simulink model "cst_robotarm_optimized"  (R2024b)
settings: Solver=ode23t  StartTime=0.0  StopTime=5  FixedStep=0.0001  MaxStep=0.05  RelTol=1e-3  EnableMultiTasking=on
model workspace (MAT data in the model file):
  DCMotor_J = 0.0946866703633
  DCMotor_K = 0.477771340295
  DCMotor_Kf = 0.921434142151
  DCMotor_L = 0.000316454712175
  DCMotor_R = 4.99938152603
  Ts = 0.1
  dFilt = [1 -0.1202]
  nFilt = [0.4399 0.4399]
values from neighbouring files (symbols this model uses):
  m = s(1)    [PIDOptimizer.m]    (also in cost.m; cost_adapted.m; cost_adopted.m)
  s = size(signals)    [PIDOptimizer.m]    (also in cost.m; cost_adapted.m; cost_adopted.m)
undefined symbols (not defined in the file or in its folder): joint1_ctrl, joint2_ctrl, joint3_ctrl, joint4_ctrl, joint5_ctrl, joint6_ctrl, X, Y, Z
libraries: sm_lib x244, fl_lib x75, nesl_utility x28, ee_lib x21, slpidlib x6, SignalEditorBlockLib x1
(part 1 of 7)
settings Model: SimulationMode=accelerator  Creator=The MathWorks, Inc.  LastModifiedBy=sergi
settings SolverCC: AlgebraicLoopSolver=TrustRegion
settings DataIOCC: LimitDataPoints=on  SaveFormat=Array  InspectSignalLogs=on  SaveTime=off  ReturnWorkspaceOutputs=off
settings OptimizationCC: ReuseModelBlockBuffer=off  ExpressionDepthLimit=2147483647  LifeSpan=inf
settings DebuggingCC: UnderspecifiedInitializationDetection=Classic  MergeDetectMultiDrivingBlocksExec=none  FcnCallInpInsideContextMsg=warning  UnconnectedInputMsg=warning  UnconnectedOutputMsg=warning  UnconnectedLineMsg=warning  StateNameClashWarn=warning  SFUnexpectedBacktrackingDiag=warning  SFNoUnconditionalDefaultTransitionDiag=warning  SFExecutionAtInitializationDiag=none  ArithmeticOperatorsInVariantConditions=warning
settings HardwareCC: ProdBitPerPointer=32  ProdBitPerSizeT=32  ProdBitPerPtrDiffT=32  ProdLargestAtomicFloat=None  ProdIntDivRoundTo=Undefined  ProdEndianess=Unspecified  ProdWordSize=32  ProdHWDeviceType=32-bit Generic
settings ModelReferenceCC: EnableRefExpFcnMdlSchedulingChecks=on  PropagateSignalLabelsOutOfModel=off
settings SFSimCC: SimUseLocalCustomCode=off  CustomCodeUndefinedFunction=UseInterfaceOnly
settings RTWCC: RTWUseLocalCustomCode=off  GPUComputeCapability=3.5
settings CodeAppCC: StateflowObjectComments=on
settings GRTTargetCC: TargetLangStandard=C89/C90 (ANSI)  CombineOutputUpdateFcns=off  GRTInterface=on
settings ConfigComp: CovMetricSettings=dw  CovSaveCumulativeToWorkspaceVar=on  CovSaveSingleToWorkspaceVar=on  CovExternalEMLEnable=off  CovSFcnEnable=off
settings SimscapeCC: SimscapeNormalizeSystem=off
settings ConfigurationSet: Description=SimMechanics 2G
settings DiagnosticsConfigSet: SimMechanicsUnconnectedFramePorts=none
settings ExplorerConfigSet: InternalSimMechanicsExplorerSettings="<ExplorerConfiguration><canonicalview>planar_xy</canonicalview><AnimationSetting><BasePlaybackSpeed>1.0</BasePlaybackSpeed><PlaybackSpeedFactor>1.0</PlaybackSpeedFactor></AnimationSetting><TilePanel><TileInfo><Tiles Columns=\"1\" Count=\"1\" Rows=\"1\"><Column Left=\"2\" Weight=\"1\"/><Column Left=\"708\"/><Row Top=\"2\" Weight=\"1\"/><Row Top=\"595\"/><Tile Height=\"1\" Width=\"1\" X=\"0\" Y=\"0\"/></Tiles></TileInfo><SceneInfo><SceneViewer><BGColor><R>0.80000001192092896</R><G>0.80000001192092896</G><B>0.80000001192092896</B></BGColor><Camera><Position><X>0.30752487944302698</X><Y>0.57922836563106395</Y><Z>0.35651305744246536</Z></Position><Center><X>-0.033772386749033274</X><Y>0.23793109943898419</Y><Z>0.015215791250393121</Z></Center><Up><X>-0.40824829046386307</X><Y>0.81649658092772615</Y><Z>-0.40824829046386307</Z></Up><Left>-0.063283674940751766</Left><Right>0.063283674940751766</Right><Bottom>-0.22321517040744418</Bottom><Top>0.22321517040744418</Top></Camera></SceneViewer></SceneInfo></TilePanel></ExplorerConfiguration>"

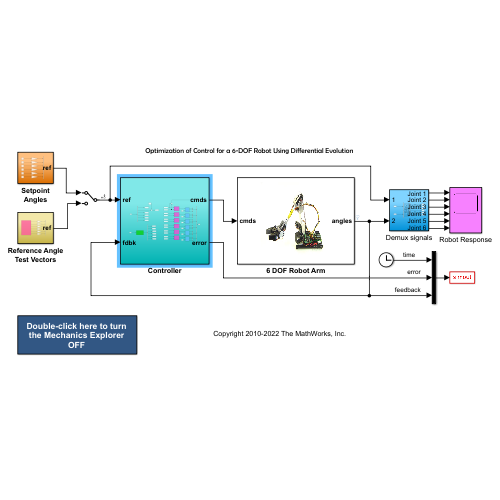
[thumbnail: Simulink's stored preview of the top-level diagram]
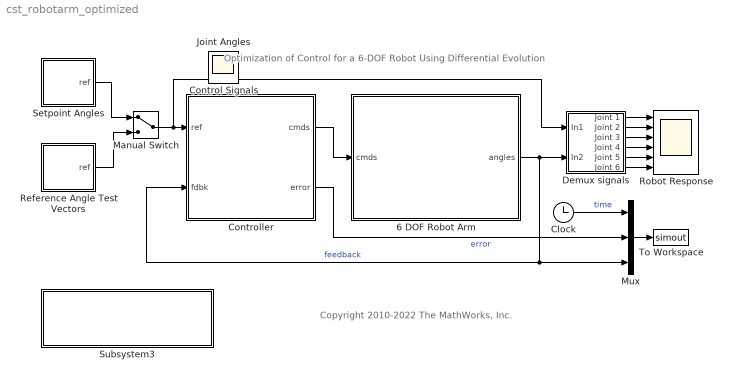
== system cst_robotarm_optimized ==
  note: Optimization of Control for a 6-DOF Robot Using Differential Evolution
  note: Copyright 2010-2022 The MathWorks, Inc.
  6 DOF Robot Arm : Subsystem
      mask Display: image('RobotArmSystem.jpg',[0.2 0.05 0.6 0.9])
  Clock : Clock
  Controller : Subsystem
  Demux signals : Subsystem
  Manual Switch : ManualSwitch
  Mux : Mux  Inputs=3
  Reference Angle Test Vectors : Subsystem
  Robot Response : Scope  NumInputPorts=6
  Setpoint Angles : Subsystem
  Subsystem3 : Subsystem
      mask init:
      | % Get current simulation mode
      | vizStatus = get_param(gcs,'SimMechanicsOpenEditorOnUpdate');
      | 
      | if strcmp(vizStatus,'on')
      |     viz = 'OFF';
      | else
      |     viz = 'ON';
      | end
      settings: OpenFcn=|
      | % Get current SimMechanics Explorer status
      | vizStatus = get_param(gcs ,'SimMechanicsOpenEditorOnUpdate');
      | 
      | if strcmp(vizStatus,'on')
      | % Set SimMechanics Explorer status to OFF
      |      set_param(gcs,'SimMechanicsOpenEditorOnUpdate','off');
      |      set_param(gcb,'BackgroundColor','[0.4706, 0.4706, 0.4706]');
      |      set_param(gcs,'SimulationCommand','update');
      | else
      | % Set SimMechanics Explorer status to ON
      |      set_param(gcs,'SimMechanicsOpenEditorOnUpdate','on');
      |      set_param(gcb,'BackgroundColor','[0.1961, 0.3412, 0.5176]')
      |      set_param(gcs,'SimulationCommand','update');
      | end
      mask Display:
      | color('white')
      | text(0.5,0.65,'Double-click here to turn\nthe Mechanics Explorer',...
      |     'horizontalAlignment','center',...
      |     'verticalAlignment','middle');
      | text(0.5,0.25,viz,...
      |     'horizontalAlignment','center',...
      |     'verticalAlignment','middle')
  To Workspace : ToWorkspace  VariableName=simout  SaveFormat=Structure With Time  SampleTime=-1
  Control Signals : Scope
  Joint Angles : Scope
  wires:
  Controller/1(cmds) -> 6 DOF Robot Arm/1(cmds)
  Manual Switch/1 -> Demux signals/1(In1), Controller/1(ref)
  Reference Angle Test Vectors/1(ref) -> Manual Switch/2
  Setpoint Angles/1(ref) -> Manual Switch/1
  Mux/1 -> To Workspace/1
  Clock/1 -> Mux/1  "time"
  6 DOF Robot Arm/1(angles) -> Mux/3, Controller/2(fdbk), Demux signals/2(In2)  "feedback"
  Controller/2(error) -> Mux/2  "error"
  Demux signals/1(Joint 1) -> Robot Response/1
  Demux signals/2(Joint 2) -> Robot Response/2
  Demux signals/3(Joint 3) -> Robot Response/3
  Demux signals/4(Joint 4) -> Robot Response/4
  Demux signals/5(Joint 5) -> Robot Response/5
  Demux signals/6(Joint 6) -> Robot Response/6

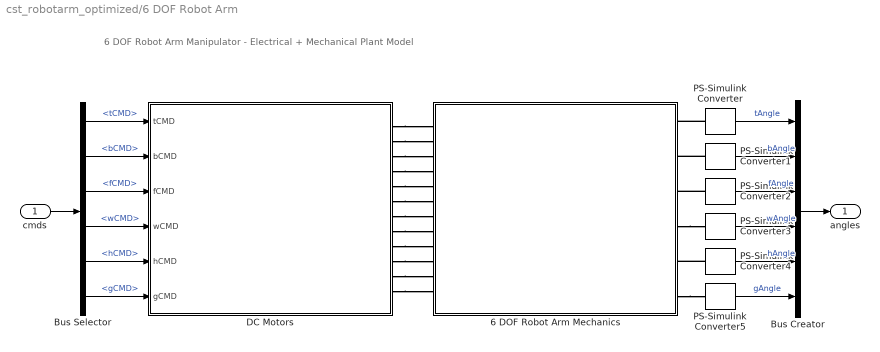
== system cst_robotarm_optimized/6 DOF Robot Arm ==
  note: 6 DOF Robot Arm Manipulator - Electrical + Mechanical Plant Model
  cmds : Inport
  6 DOF Robot Arm Mechanics : Subsystem
      mask Display: image('RobotArm_Mechanics.jpg',[0.1 0 0.8 1])
  Bus Creator : BusCreator  Inputs=6
  Bus Selector : BusSelector  OutputSignals=tCMD,bCMD,fCMD,wCMD,hCMD,gCMD
  DC Motors : Subsystem
      mask Display: image('MultiServos.jpg',[0.25 0.1 0.5 0.8])
  PS-Simulink Converter{,1..5} (6 alike) : nesl_utility/PS-Simulink Converter  PhysicalDomain=network_engine_domain  SubClassName=ps_output  LeftPortType=input  RightPortType=output  PseudoPeriodic=off  Frequencies=[]  VectorFormat=1-D array  Unit=rad  AffineConversion=off
  angles : Outport  VectorParamsAs1DForOutWhenUnconnected=off
  wires:
  Bus Creator/1 -> angles/1
  PS-Simulink Converter2/1 -> Bus Creator/3  "fAngle"
  PS-Simulink Converter5/1 -> Bus Creator/6  "gAngle"
  PS-Simulink Converter/1 -> Bus Creator/1  "tAngle"
  PS-Simulink Converter1/1 -> Bus Creator/2  "bAngle"
  PS-Simulink Converter3/1 -> Bus Creator/4  "wAngle"
  PS-Simulink Converter4/1 -> Bus Creator/5  "hAngle"
  Bus Selector/6 -> DC Motors/6(gCMD)  "<gCMD>"
  Bus Selector/3 -> DC Motors/3(fCMD)  "<fCMD>"
  Bus Selector/4 -> DC Motors/4(wCMD)  "<wCMD>"
  Bus Selector/2 -> DC Motors/2(bCMD)  "<bCMD>"
  Bus Selector/5 -> DC Motors/5(hCMD)  "<hCMD>"
  Bus Selector/1 -> DC Motors/1(tCMD)  "<tCMD>"
  cmds/1 -> Bus Selector/1
  connections:
  PS-Simulink Converter2/LConn1 -- 6 DOF Robot Arm Mechanics/RConn3
  DC Motors/RConn7 -- 6 DOF Robot Arm Mechanics/LConn7
  DC Motors/RConn8 -- 6 DOF Robot Arm Mechanics/LConn8
  DC Motors/RConn6 -- 6 DOF Robot Arm Mechanics/LConn6
  PS-Simulink Converter/LConn1 -- 6 DOF Robot Arm Mechanics/RConn1
  DC Motors/RConn2 -- 6 DOF Robot Arm Mechanics/LConn2
  DC Motors/RConn5 -- 6 DOF Robot Arm Mechanics/LConn5
  DC Motors/RConn11 -- 6 DOF Robot Arm Mechanics/LConn11
  DC Motors/RConn12 -- 6 DOF Robot Arm Mechanics/LConn12
  DC Motors/RConn9 -- 6 DOF Robot Arm Mechanics/LConn9
  DC Motors/RConn3 -- 6 DOF Robot Arm Mechanics/LConn3
  DC Motors/RConn4 -- 6 DOF Robot Arm Mechanics/LConn4
  PS-Simulink Converter1/LConn1 -- 6 DOF Robot Arm Mechanics/RConn2
  PS-Simulink Converter4/LConn1 -- 6 DOF Robot Arm Mechanics/RConn5
  6 DOF Robot Arm Mechanics/RConn6 -- PS-Simulink Converter5/LConn1
  6 DOF Robot Arm Mechanics/RConn4 -- PS-Simulink Converter3/LConn1
  DC Motors/RConn10 -- 6 DOF Robot Arm Mechanics/LConn10
  DC Motors/RConn1 -- 6 DOF Robot Arm Mechanics/LConn1

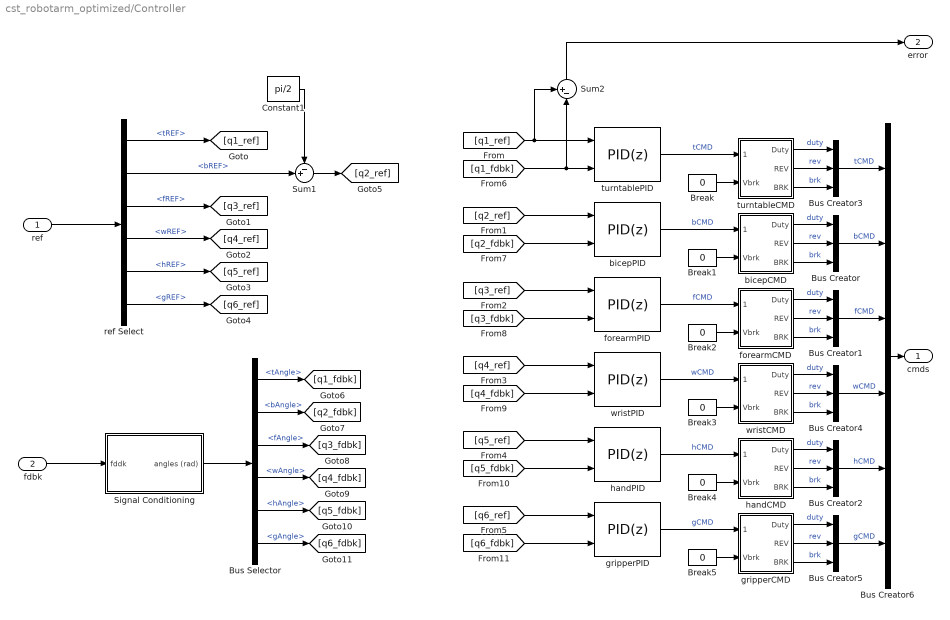
== system cst_robotarm_optimized/Controller ==
  ref : Inport
  fdbk : Inport  Port=2
  Break{,1..5} (6 alike) : Constant  Value=0
  Bus Creator{,1..5} (6 alike) : BusCreator  Inputs=3
  Bus Creator6 : BusCreator  Inputs=6
  Bus Selector : BusSelector  OutputSignals=tAngle,bAngle,fAngle,wAngle,hAngle,gAngle
  Constant1 : Constant  Value=pi/2
  Signal Conditioning : Subsystem
  Sum1 : Sum  Inputs=-+|
  Sum2 : Sum  Inputs=+-|
  bicepCMD : Subsystem
  bicepPID : slpidlib/PID Controller (2DOF)  Controller=PID  Form=Parallel  TimeDomain=Discrete-time  UseExternalTs=off  SampleTime=Ts  IntegratorMethod=Forward Euler  FilterMethod=Backward Euler  ControllerParametersSource=internal  P=17.9852  I=20.5596  UseKiTs=off  D=0  UseExternalDerivativeSource=off  N=25  UseFilter=on  b=1  c=1  TunerSelectOption=Transfer Function Based (PID Tuner App)  InitialConditionSource=internal  InitialConditionForIntegrator=0  InitialConditionForFilter=0  DifferentiatorICPrevScaledInput=0  ExternalReset=none  TrackingMode=off  Kt=1  LimitOutput=on  SatLimitsSource=internal  UpperSaturationLimit=5  LowerSaturationLimit=-5  LinearizeAsGain=on  AntiWindupMode=clamping  Kb=1  LimitIntegrator=off  UpperIntegratorSaturationLimit=inf  LowerIntegratorSaturationLimit=-inf  POutMin=[]  POutMax=[]  IOutMin=[]  IOutMax=[]  DOutMin=[]  DOutMax=[]  NOutMin=[]  NOutMax=[]  bOutMin=[]  bOutMax=[]  cOutMin=[]  cOutMax=[]  SumOutMin=[]  SumOutMax=[]  SaturationOutMin=[]  SaturationOutMax=[]  PParamMin=[]  PParamMax=[]  IParamMin=[]  IParamMax=[]  DParamMin=[]  DParamMax=[]  NParamMin=[]  NParamMax=[]  bParamMin=[]  bParamMax=[]  cParamMin=[]  cParamMax=[]  KbParamMin=[]  KbParamMax=[]  KtParamMin=[]  KtParamMax=[]  KbOutMin=[]  KbOutMax=[]  KtOutMin=[]  KtOutMax=[]  IntegratorOutMin=[]  IntegratorOutMax=[]  FilterOutMin=[]  FilterOutMax=[]  SumI1OutMin=[]  SumI1OutMax=[]  SumI2OutMin=[]  SumI2OutMax=[]  SumI3OutMin=[]  SumI3OutMax=[]  SumI4OutMin=[]  SumI4OutMax=[]  SumDOutMin=[]  SumDOutMax=[]  Sum1OutMin=[]  Sum1OutMax=[]  Sum2OutMin=[]  Sum2OutMax=[]  Sum3OutMin=[]  Sum3OutMax=[]  DifferentiatorOutMin=[]  DifferentiatorOutMax=[]  FilterDiffOutCoefMin=[]  FilterDiffOutCoefMax=[]  ReciprocalOutMin=[]  ReciprocalOutMax=[]  SumDenOutMin=[]  SumDenOutMax=[]  SumNumOutMin=[]  SumNumOutMax=[]  DivideOutMin=[]  DivideOutMax=[]  UdiffTsProdOutMin=[]  UdiffTsProdOutMax=[]  NTsProdOutMin=[]  NTsProdOutMax=[]  UintegralTsProdOutMin=[]  UintegralTsProdOutMax=[]  UngainTsProdOutMin=[]  UngainTsProdOutMax=[]  ClampingZeroOutDataTypeStr=Inherit: Inherit via back propagation  ClampingZeroOutMin=[]  ClampingZeroOutMax=[]  FilterDenConstantOutDataTypeStr=Inherit: Inherit via back propagation  FilterDenConstantOutMin=[]  FilterDenConstantOutMax=[]  PCopyOutDataTypeStr=Inherit: Inherit via back propagation  PCopyOutMin=[]  PCopyOutMax=[]  NCopyOutDataTypeStr=Inherit: Inherit via back propagation  NCopyOutMin=[]  NCopyOutMax=[]  IntegratorContinuousStateAttributes=''  IntegratorStateMustResolveToSignalObject=off  IntegratorRTWStateStorageClass=Auto  FilterContinuousStateAttributes=''  FilterStateMustResolveToSignalObject=off  FilterRTWStateStorageClass=Auto  ParallelPVariant=InternalParameters  IdealPVariant=Disabled  IVariant=InternalParameters  DVariant=InternalParameters  bVariant=InternalParameters  cVariant=InternalParameters  IntegratorVariant=Discrete  SatVariant=Enabled  AWVariant=DiscClampingParallel  PCopyVariant=Disabled  TRVariant=Disabled  FdbkBlocksVariant=Forward  IdealPFdbkVariant=Disabled  SatFdbkVariant=Disabled  DerivativeFilterVariant=BackwardEulerFilter  NVariant=InternalParameters  NCopyVariant=InternalParameters  FilterICVariant=InternalICsFilter  IntegratorICVariant=InternalICs  ExternalResetVariant=Disabled  TRSumVariant=Passthrough  SumFdbkVariant=Disabled  SumVariant=Sum_PID  TsampFilterVariant=InternalTs  TsampNgainVariant=Passthrough  TsampIntegralVariant=Disabled_SignalSpec  ExternalSaturationOutDataTypeStr=Inherit: Same as second input  DerivativeSourceVariant=ErrorSignal  PreIntVariant=InternalPreInt
  forearmCMD : Subsystem
  forearmPID : slpidlib/PID Controller (2DOF)  Controller=PID  Form=Parallel  TimeDomain=Discrete-time  UseExternalTs=off  SampleTime=Ts  IntegratorMethod=Forward Euler  FilterMethod=Backward Euler  ControllerParametersSource=internal  P=9.2892  I=16.8208  UseKiTs=off  D=0.0153  UseExternalDerivativeSource=off  N=25  UseFilter=on  b=1  c=1  TunerSelectOption=Transfer Function Based (PID Tuner App)  InitialConditionSource=internal  InitialConditionForIntegrator=0  InitialConditionForFilter=0  DifferentiatorICPrevScaledInput=0  ExternalReset=none  TrackingMode=off  Kt=1  LimitOutput=on  SatLimitsSource=internal  UpperSaturationLimit=5  LowerSaturationLimit=-5  LinearizeAsGain=on  AntiWindupMode=clamping  Kb=1  LimitIntegrator=off  UpperIntegratorSaturationLimit=inf  LowerIntegratorSaturationLimit=-inf  POutMin=[]  POutMax=[]  IOutMin=[]  IOutMax=[]  DOutMin=[]  DOutMax=[]  NOutMin=[]  NOutMax=[]  bOutMin=[]  bOutMax=[]  cOutMin=[]  cOutMax=[]  SumOutMin=[]  SumOutMax=[]  SaturationOutMin=[]  SaturationOutMax=[]  PParamMin=[]  PParamMax=[]  IParamMin=[]  IParamMax=[]  DParamMin=[]  DParamMax=[]  NParamMin=[]  NParamMax=[]  bParamMin=[]  bParamMax=[]  cParamMin=[]  cParamMax=[]  KbParamMin=[]  KbParamMax=[]  KtParamMin=[]  KtParamMax=[]  KbOutMin=[]  KbOutMax=[]  KtOutMin=[]  KtOutMax=[]  IntegratorOutMin=[]  IntegratorOutMax=[]  FilterOutMin=[]  FilterOutMax=[]  SumI1OutMin=[]  SumI1OutMax=[]  SumI2OutMin=[]  SumI2OutMax=[]  SumI3OutMin=[]  SumI3OutMax=[]  SumI4OutMin=[]  SumI4OutMax=[]  SumDOutMin=[]  SumDOutMax=[]  Sum1OutMin=[]  Sum1OutMax=[]  Sum2OutMin=[]  Sum2OutMax=[]  Sum3OutMin=[]  Sum3OutMax=[]  DifferentiatorOutMin=[]  DifferentiatorOutMax=[]  FilterDiffOutCoefMin=[]  FilterDiffOutCoefMax=[]  ReciprocalOutMin=[]  ReciprocalOutMax=[]  SumDenOutMin=[]  SumDenOutMax=[]  SumNumOutMin=[]  SumNumOutMax=[]  DivideOutMin=[]  DivideOutMax=[]  UdiffTsProdOutMin=[]  UdiffTsProdOutMax=[]  NTsProdOutMin=[]  NTsProdOutMax=[]  UintegralTsProdOutMin=[]  UintegralTsProdOutMax=[]  UngainTsProdOutMin=[]  UngainTsProdOutMax=[]  ClampingZeroOutDataTypeStr=Inherit: Inherit via back propagation  ClampingZeroOutMin=[]  ClampingZeroOutMax=[]  FilterDenConstantOutDataTypeStr=Inherit: Inherit via back propagation  FilterDenConstantOutMin=[]  FilterDenConstantOutMax=[]  PCopyOutDataTypeStr=Inherit: Inherit via back propagation  PCopyOutMin=[]  PCopyOutMax=[]  NCopyOutDataTypeStr=Inherit: Inherit via back propagation  NCopyOutMin=[]  NCopyOutMax=[]  IntegratorContinuousStateAttributes=''  IntegratorStateMustResolveToSignalObject=off  IntegratorRTWStateStorageClass=Auto  FilterContinuousStateAttributes=''  FilterStateMustResolveToSignalObject=off  FilterRTWStateStorageClass=Auto  ParallelPVariant=InternalParameters  IdealPVariant=Disabled  IVariant=InternalParameters  DVariant=InternalParameters  bVariant=InternalParameters  cVariant=InternalParameters  IntegratorVariant=Discrete  SatVariant=Enabled  AWVariant=DiscClampingParallel  PCopyVariant=Disabled  TRVariant=Disabled  FdbkBlocksVariant=Forward  IdealPFdbkVariant=Disabled  SatFdbkVariant=Disabled  DerivativeFilterVariant=BackwardEulerFilter  NVariant=InternalParameters  NCopyVariant=InternalParameters  FilterICVariant=InternalICsFilter  IntegratorICVariant=InternalICs  ExternalResetVariant=Disabled  TRSumVariant=Passthrough  SumFdbkVariant=Disabled  SumVariant=Sum_PID  TsampFilterVariant=InternalTs  TsampNgainVariant=Passthrough  TsampIntegralVariant=Disabled_SignalSpec  ExternalSaturationOutDataTypeStr=Inherit: Same as second input  DerivativeSourceVariant=ErrorSignal  PreIntVariant=InternalPreInt
  gripperCMD : Subsystem
  gripperPID : slpidlib/PID Controller (2DOF)  Controller=PID  Form=Parallel  TimeDomain=Discrete-time  UseExternalTs=off  SampleTime=Ts  IntegratorMethod=Forward Euler  FilterMethod=Backward Euler  ControllerParametersSource=internal  P=14.2833  I=0  UseKiTs=off  D=0  UseExternalDerivativeSource=off  N=25  UseFilter=on  b=1  c=1  TunerSelectOption=Transfer Function Based (PID Tuner App)  InitialConditionSource=internal  InitialConditionForIntegrator=0  InitialConditionForFilter=0  DifferentiatorICPrevScaledInput=0  ExternalReset=none  TrackingMode=off  Kt=1  LimitOutput=on  SatLimitsSource=internal  UpperSaturationLimit=5  LowerSaturationLimit=-5  LinearizeAsGain=on  AntiWindupMode=clamping  Kb=1  LimitIntegrator=off  UpperIntegratorSaturationLimit=inf  LowerIntegratorSaturationLimit=-inf  POutMin=[]  POutMax=[]  IOutMin=[]  IOutMax=[]  DOutMin=[]  DOutMax=[]  NOutMin=[]  NOutMax=[]  bOutMin=[]  bOutMax=[]  cOutMin=[]  cOutMax=[]  SumOutMin=[]  SumOutMax=[]  SaturationOutMin=[]  SaturationOutMax=[]  PParamMin=[]  PParamMax=[]  IParamMin=[]  IParamMax=[]  DParamMin=[]  DParamMax=[]  NParamMin=[]  NParamMax=[]  bParamMin=[]  bParamMax=[]  cParamMin=[]  cParamMax=[]  KbParamMin=[]  KbParamMax=[]  KtParamMin=[]  KtParamMax=[]  KbOutMin=[]  KbOutMax=[]  KtOutMin=[]  KtOutMax=[]  IntegratorOutMin=[]  IntegratorOutMax=[]  FilterOutMin=[]  FilterOutMax=[]  SumI1OutMin=[]  SumI1OutMax=[]  SumI2OutMin=[]  SumI2OutMax=[]  SumI3OutMin=[]  SumI3OutMax=[]  SumI4OutMin=[]  SumI4OutMax=[]  SumDOutMin=[]  SumDOutMax=[]  Sum1OutMin=[]  Sum1OutMax=[]  Sum2OutMin=[]  Sum2OutMax=[]  Sum3OutMin=[]  Sum3OutMax=[]  DifferentiatorOutMin=[]  DifferentiatorOutMax=[]  FilterDiffOutCoefMin=[]  FilterDiffOutCoefMax=[]  ReciprocalOutMin=[]  ReciprocalOutMax=[]  SumDenOutMin=[]  SumDenOutMax=[]  SumNumOutMin=[]  SumNumOutMax=[]  DivideOutMin=[]  DivideOutMax=[]  UdiffTsProdOutMin=[]  UdiffTsProdOutMax=[]  NTsProdOutMin=[]  NTsProdOutMax=[]  UintegralTsProdOutMin=[]  UintegralTsProdOutMax=[]  UngainTsProdOutMin=[]  UngainTsProdOutMax=[]  ClampingZeroOutDataTypeStr=Inherit: Inherit via back propagation  ClampingZeroOutMin=[]  ClampingZeroOutMax=[]  FilterDenConstantOutDataTypeStr=Inherit: Inherit via back propagation  FilterDenConstantOutMin=[]  FilterDenConstantOutMax=[]  PCopyOutDataTypeStr=Inherit: Inherit via back propagation  PCopyOutMin=[]  PCopyOutMax=[]  NCopyOutDataTypeStr=Inherit: Inherit via back propagation  NCopyOutMin=[]  NCopyOutMax=[]  IntegratorContinuousStateAttributes=''  IntegratorStateMustResolveToSignalObject=off  IntegratorRTWStateStorageClass=Auto  FilterContinuousStateAttributes=''  FilterStateMustResolveToSignalObject=off  FilterRTWStateStorageClass=Auto  ParallelPVariant=InternalParameters  IdealPVariant=Disabled  IVariant=InternalParameters  DVariant=InternalParameters  bVariant=InternalParameters  cVariant=InternalParameters  IntegratorVariant=Discrete  SatVariant=Enabled  AWVariant=DiscClampingParallel  PCopyVariant=Disabled  TRVariant=Disabled  FdbkBlocksVariant=Forward  IdealPFdbkVariant=Disabled  SatFdbkVariant=Disabled  DerivativeFilterVariant=BackwardEulerFilter  NVariant=InternalParameters  NCopyVariant=InternalParameters  FilterICVariant=InternalICsFilter  IntegratorICVariant=InternalICs  ExternalResetVariant=Disabled  TRSumVariant=Passthrough  SumFdbkVariant=Disabled  SumVariant=Sum_PID  TsampFilterVariant=InternalTs  TsampNgainVariant=Passthrough  TsampIntegralVariant=Disabled_SignalSpec  ExternalSaturationOutDataTypeStr=Inherit: Same as second input  DerivativeSourceVariant=ErrorSignal  PreIntVariant=InternalPreInt
  handCMD : Subsystem
  handPID : slpidlib/PID Controller (2DOF)  Controller=PID  Form=Parallel  TimeDomain=Discrete-time  UseExternalTs=off  SampleTime=Ts  IntegratorMethod=Forward Euler  FilterMethod=Backward Euler  ControllerParametersSource=internal  P=12.3126  I=0.1702  UseKiTs=off  D=0  UseExternalDerivativeSource=off  N=25  UseFilter=on  b=1  c=1  TunerSelectOption=Transfer Function Based (PID Tuner App)  InitialConditionSource=internal  InitialConditionForIntegrator=0  InitialConditionForFilter=0  DifferentiatorICPrevScaledInput=0  ExternalReset=none  TrackingMode=off  Kt=1  LimitOutput=on  SatLimitsSource=internal  UpperSaturationLimit=5  LowerSaturationLimit=-5  LinearizeAsGain=on  AntiWindupMode=clamping  Kb=1  LimitIntegrator=off  UpperIntegratorSaturationLimit=inf  LowerIntegratorSaturationLimit=-inf  POutMin=[]  POutMax=[]  IOutMin=[]  IOutMax=[]  DOutMin=[]  DOutMax=[]  NOutMin=[]  NOutMax=[]  bOutMin=[]  bOutMax=[]  cOutMin=[]  cOutMax=[]  SumOutMin=[]  SumOutMax=[]  SaturationOutMin=[]  SaturationOutMax=[]  PParamMin=[]  PParamMax=[]  IParamMin=[]  IParamMax=[]  DParamMin=[]  DParamMax=[]  NParamMin=[]  NParamMax=[]  bParamMin=[]  bParamMax=[]  cParamMin=[]  cParamMax=[]  KbParamMin=[]  KbParamMax=[]  KtParamMin=[]  KtParamMax=[]  KbOutMin=[]  KbOutMax=[]  KtOutMin=[]  KtOutMax=[]  IntegratorOutMin=[]  IntegratorOutMax=[]  FilterOutMin=[]  FilterOutMax=[]  SumI1OutMin=[]  SumI1OutMax=[]  SumI2OutMin=[]  SumI2OutMax=[]  SumI3OutMin=[]  SumI3OutMax=[]  SumI4OutMin=[]  SumI4OutMax=[]  SumDOutMin=[]  SumDOutMax=[]  Sum1OutMin=[]  Sum1OutMax=[]  Sum2OutMin=[]  Sum2OutMax=[]  Sum3OutMin=[]  Sum3OutMax=[]  DifferentiatorOutMin=[]  DifferentiatorOutMax=[]  FilterDiffOutCoefMin=[]  FilterDiffOutCoefMax=[]  ReciprocalOutMin=[]  ReciprocalOutMax=[]  SumDenOutMin=[]  SumDenOutMax=[]  SumNumOutMin=[]  SumNumOutMax=[]  DivideOutMin=[]  DivideOutMax=[]  UdiffTsProdOutMin=[]  UdiffTsProdOutMax=[]  NTsProdOutMin=[]  NTsProdOutMax=[]  UintegralTsProdOutMin=[]  UintegralTsProdOutMax=[]  UngainTsProdOutMin=[]  UngainTsProdOutMax=[]  ClampingZeroOutDataTypeStr=Inherit: Inherit via back propagation  ClampingZeroOutMin=[]  ClampingZeroOutMax=[]  FilterDenConstantOutDataTypeStr=Inherit: Inherit via back propagation  FilterDenConstantOutMin=[]  FilterDenConstantOutMax=[]  PCopyOutDataTypeStr=Inherit: Inherit via back propagation  PCopyOutMin=[]  PCopyOutMax=[]  NCopyOutDataTypeStr=Inherit: Inherit via back propagation  NCopyOutMin=[]  NCopyOutMax=[]  IntegratorContinuousStateAttributes=''  IntegratorStateMustResolveToSignalObject=off  IntegratorRTWStateStorageClass=Auto  FilterContinuousStateAttributes=''  FilterStateMustResolveToSignalObject=off  FilterRTWStateStorageClass=Auto  ParallelPVariant=InternalParameters  IdealPVariant=Disabled  IVariant=InternalParameters  DVariant=InternalParameters  bVariant=InternalParameters  cVariant=InternalParameters  IntegratorVariant=Discrete  SatVariant=Enabled  AWVariant=DiscClampingParallel  PCopyVariant=Disabled  TRVariant=Disabled  FdbkBlocksVariant=Forward  IdealPFdbkVariant=Disabled  SatFdbkVariant=Disabled  DerivativeFilterVariant=BackwardEulerFilter  NVariant=InternalParameters  NCopyVariant=InternalParameters  FilterICVariant=InternalICsFilter  IntegratorICVariant=InternalICs  ExternalResetVariant=Disabled  TRSumVariant=Passthrough  SumFdbkVariant=Disabled  SumVariant=Sum_PID  TsampFilterVariant=InternalTs  TsampNgainVariant=Passthrough  TsampIntegralVariant=Disabled_SignalSpec  ExternalSaturationOutDataTypeStr=Inherit: Same as second input  DerivativeSourceVariant=ErrorSignal  PreIntVariant=InternalPreInt
  ref Select : BusSelector  OutputSignals=tREF,bREF,fREF,wREF,hREF,gREF
  turntableCMD : Subsystem
  turntablePID : slpidlib/PID Controller (2DOF)  Controller=PID  Form=Parallel  TimeDomain=Discrete-time  UseExternalTs=off  SampleTime=Ts  IntegratorMethod=Forward Euler  FilterMethod=Backward Euler  ControllerParametersSource=internal  P=11.8483  I=0.1859  UseKiTs=off  D=0.0039  UseExternalDerivativeSource=off  N=25  UseFilter=on  b=1  c=1  TunerSelectOption=Transfer Function Based (PID Tuner App)  InitialConditionSource=internal  InitialConditionForIntegrator=0  InitialConditionForFilter=0  DifferentiatorICPrevScaledInput=0  ExternalReset=none  TrackingMode=off  Kt=1  LimitOutput=on  SatLimitsSource=internal  UpperSaturationLimit=5  LowerSaturationLimit=-5  LinearizeAsGain=on  AntiWindupMode=clamping  Kb=1  LimitIntegrator=off  UpperIntegratorSaturationLimit=inf  LowerIntegratorSaturationLimit=-inf  POutMin=[]  POutMax=[]  IOutMin=[]  IOutMax=[]  DOutMin=[]  DOutMax=[]  NOutMin=[]  NOutMax=[]  bOutMin=[]  bOutMax=[]  cOutMin=[]  cOutMax=[]  SumOutMin=[]  SumOutMax=[]  SaturationOutMin=[]  SaturationOutMax=[]  PParamMin=[]  PParamMax=[]  IParamMin=[]  IParamMax=[]  DParamMin=[]  DParamMax=[]  NParamMin=[]  NParamMax=[]  bParamMin=[]  bParamMax=[]  cParamMin=[]  cParamMax=[]  KbParamMin=[]  KbParamMax=[]  KtParamMin=[]  KtParamMax=[]  KbOutMin=[]  KbOutMax=[]  KtOutMin=[]  KtOutMax=[]  IntegratorOutMin=[]  IntegratorOutMax=[]  FilterOutMin=[]  FilterOutMax=[]  SumI1OutMin=[]  SumI1OutMax=[]  SumI2OutMin=[]  SumI2OutMax=[]  SumI3OutMin=[]  SumI3OutMax=[]  SumI4OutMin=[]  SumI4OutMax=[]  SumDOutMin=[]  SumDOutMax=[]  Sum1OutMin=[]  Sum1OutMax=[]  Sum2OutMin=[]  Sum2OutMax=[]  Sum3OutMin=[]  Sum3OutMax=[]  DifferentiatorOutMin=[]  DifferentiatorOutMax=[]  FilterDiffOutCoefMin=[]  FilterDiffOutCoefMax=[]  ReciprocalOutMin=[]  ReciprocalOutMax=[]  SumDenOutMin=[]  SumDenOutMax=[]  SumNumOutMin=[]  SumNumOutMax=[]  DivideOutMin=[]  DivideOutMax=[]  UdiffTsProdOutMin=[]  UdiffTsProdOutMax=[]  NTsProdOutMin=[]  NTsProdOutMax=[]  UintegralTsProdOutMin=[]  UintegralTsProdOutMax=[]  UngainTsProdOutMin=[]  UngainTsProdOutMax=[]  ClampingZeroOutDataTypeStr=Inherit: Inherit via back propagation  ClampingZeroOutMin=[]  ClampingZeroOutMax=[]  FilterDenConstantOutDataTypeStr=Inherit: Inherit via back propagation  FilterDenConstantOutMin=[]  FilterDenConstantOutMax=[]  PCopyOutDataTypeStr=Inherit: Inherit via back propagation  PCopyOutMin=[]  PCopyOutMax=[]  NCopyOutDataTypeStr=Inherit: Inherit via back propagation  NCopyOutMin=[]  NCopyOutMax=[]  IntegratorContinuousStateAttributes=''  IntegratorStateMustResolveToSignalObject=off  IntegratorRTWStateStorageClass=Auto  FilterContinuousStateAttributes=''  FilterStateMustResolveToSignalObject=off  FilterRTWStateStorageClass=Auto  ParallelPVariant=InternalParameters  IdealPVariant=Disabled  IVariant=InternalParameters  DVariant=InternalParameters  bVariant=InternalParameters  cVariant=InternalParameters  IntegratorVariant=Discrete  SatVariant=Enabled  AWVariant=DiscClampingParallel  PCopyVariant=Disabled  TRVariant=Disabled  FdbkBlocksVariant=Forward  IdealPFdbkVariant=Disabled  SatFdbkVariant=Disabled  DerivativeFilterVariant=BackwardEulerFilter  NVariant=InternalParameters  NCopyVariant=InternalParameters  FilterICVariant=InternalICsFilter  IntegratorICVariant=InternalICs  ExternalResetVariant=Disabled  TRSumVariant=Passthrough  SumFdbkVariant=Disabled  SumVariant=Sum_PID  TsampFilterVariant=InternalTs  TsampNgainVariant=Passthrough  TsampIntegralVariant=Disabled_SignalSpec  ExternalSaturationOutDataTypeStr=Inherit: Same as second input  DerivativeSourceVariant=ErrorSignal  PreIntVariant=InternalPreInt
  wristCMD : Subsystem
  wristPID : slpidlib/PID Controller (2DOF)  Controller=PID  Form=Parallel  TimeDomain=Discrete-time  UseExternalTs=off  SampleTime=Ts  IntegratorMethod=Forward Euler  FilterMethod=Backward Euler  ControllerParametersSource=internal  P=28.6230  I=11.6376  UseKiTs=off  D=0.0637  UseExternalDerivativeSource=off  N=25  UseFilter=on  b=1  c=1  TunerSelectOption=Transfer Function Based (PID Tuner App)  InitialConditionSource=internal  InitialConditionForIntegrator=0  InitialConditionForFilter=0  DifferentiatorICPrevScaledInput=0  ExternalReset=none  TrackingMode=off  Kt=1  LimitOutput=on  SatLimitsSource=internal  UpperSaturationLimit=5  LowerSaturationLimit=-5  LinearizeAsGain=on  AntiWindupMode=clamping  Kb=1  LimitIntegrator=off  UpperIntegratorSaturationLimit=inf  LowerIntegratorSaturationLimit=-inf  POutMin=[]  POutMax=[]  IOutMin=[]  IOutMax=[]  DOutMin=[]  DOutMax=[]  NOutMin=[]  NOutMax=[]  bOutMin=[]  bOutMax=[]  cOutMin=[]  cOutMax=[]  SumOutMin=[]  SumOutMax=[]  SaturationOutMin=[]  SaturationOutMax=[]  PParamMin=[]  PParamMax=[]  IParamMin=[]  IParamMax=[]  DParamMin=[]  DParamMax=[]  NParamMin=[]  NParamMax=[]  bParamMin=[]  bParamMax=[]  cParamMin=[]  cParamMax=[]  KbParamMin=[]  KbParamMax=[]  KtParamMin=[]  KtParamMax=[]  KbOutMin=[]  KbOutMax=[]  KtOutMin=[]  KtOutMax=[]  IntegratorOutMin=[]  IntegratorOutMax=[]  FilterOutMin=[]  FilterOutMax=[]  SumI1OutMin=[]  SumI1OutMax=[]  SumI2OutMin=[]  SumI2OutMax=[]  SumI3OutMin=[]  SumI3OutMax=[]  SumI4OutMin=[]  SumI4OutMax=[]  SumDOutMin=[]  SumDOutMax=[]  Sum1OutMin=[]  Sum1OutMax=[]  Sum2OutMin=[]  Sum2OutMax=[]  Sum3OutMin=[]  Sum3OutMax=[]  DifferentiatorOutMin=[]  DifferentiatorOutMax=[]  FilterDiffOutCoefMin=[]  FilterDiffOutCoefMax=[]  ReciprocalOutMin=[]  ReciprocalOutMax=[]  SumDenOutMin=[]  SumDenOutMax=[]  SumNumOutMin=[]  SumNumOutMax=[]  DivideOutMin=[]  DivideOutMax=[]  UdiffTsProdOutMin=[]  UdiffTsProdOutMax=[]  NTsProdOutMin=[]  NTsProdOutMax=[]  UintegralTsProdOutMin=[]  UintegralTsProdOutMax=[]  UngainTsProdOutMin=[]  UngainTsProdOutMax=[]  ClampingZeroOutDataTypeStr=Inherit: Inherit via back propagation  ClampingZeroOutMin=[]  ClampingZeroOutMax=[]  FilterDenConstantOutDataTypeStr=Inherit: Inherit via back propagation  FilterDenConstantOutMin=[]  FilterDenConstantOutMax=[]  PCopyOutDataTypeStr=Inherit: Inherit via back propagation  PCopyOutMin=[]  PCopyOutMax=[]  NCopyOutDataTypeStr=Inherit: Inherit via back propagation  NCopyOutMin=[]  NCopyOutMax=[]  IntegratorContinuousStateAttributes=''  IntegratorStateMustResolveToSignalObject=off  IntegratorRTWStateStorageClass=Auto  FilterContinuousStateAttributes=''  FilterStateMustResolveToSignalObject=off  FilterRTWStateStorageClass=Auto  ParallelPVariant=InternalParameters  IdealPVariant=Disabled  IVariant=InternalParameters  DVariant=InternalParameters  bVariant=InternalParameters  cVariant=InternalParameters  IntegratorVariant=Discrete  SatVariant=Enabled  AWVariant=DiscClampingParallel  PCopyVariant=Disabled  TRVariant=Disabled  FdbkBlocksVariant=Forward  IdealPFdbkVariant=Disabled  SatFdbkVariant=Disabled  DerivativeFilterVariant=BackwardEulerFilter  NVariant=InternalParameters  NCopyVariant=InternalParameters  FilterICVariant=InternalICsFilter  IntegratorICVariant=InternalICs  ExternalResetVariant=Disabled  TRSumVariant=Passthrough  SumFdbkVariant=Disabled  SumVariant=Sum_PID  TsampFilterVariant=InternalTs  TsampNgainVariant=Passthrough  TsampIntegralVariant=Disabled_SignalSpec  ExternalSaturationOutDataTypeStr=Inherit: Same as second input  DerivativeSourceVariant=ErrorSignal  PreIntVariant=InternalPreInt
  cmds : Outport  VectorParamsAs1DForOutWhenUnconnected=off
  error : Outport  Port=2
  wires:
  bicepCMD/1(Duty) -> Bus Creator/1  "duty"
  bicepCMD/2(REV) -> Bus Creator/2  "rev"
  bicepCMD/3(BRK) -> Bus Creator/3  "brk"
  forearmCMD/1(Duty) -> Bus Creator1/1  "duty"
  forearmCMD/2(REV) -> Bus Creator1/2  "rev"
  forearmCMD/3(BRK) -> Bus Creator1/3  "brk"
  handCMD/2(REV) -> Bus Creator2/2  "rev"
  handCMD/3(BRK) -> Bus Creator2/3  "brk"
  handCMD/1(Duty) -> Bus Creator2/1  "duty"
  bicepPID/1 -> bicepCMD/1(Vcmd)  "bCMD"
  Break1/1 -> bicepCMD/2(Vbrk)
  forearmPID/1 -> forearmCMD/1(Vcmd)  "fCMD"
  Break2/1 -> forearmCMD/2(Vbrk)
  handPID/1 -> handCMD/1(Vcmd)  "hCMD"
  Break4/1 -> handCMD/2(Vbrk)
  Bus Creator1/1 -> Bus Creator6/3  "fCMD"
  Bus Creator2/1 -> Bus Creator6/5  "hCMD"
  ref/1 -> ref Select/1
  turntableCMD/1(Duty) -> Bus Creator3/1  "duty"
  turntableCMD/2(REV) -> Bus Creator3/2  "rev"
  turntableCMD/3(BRK) -> Bus Creator3/3  "brk"
  turntablePID/1 -> turntableCMD/1(Vcmd)  "tCMD"
  Break/1 -> turntableCMD/2(Vbrk)
  Bus Creator3/1 -> Bus Creator6/1  "tCMD"
  wristCMD/2(REV) -> Bus Creator4/2  "rev"
  wristCMD/3(BRK) -> Bus Creator4/3  "brk"
  wristCMD/1(Duty) -> Bus Creator4/1  "duty"
  wristPID/1 -> wristCMD/1(Vcmd)  "wCMD"
  Break3/1 -> wristCMD/2(Vbrk)
  Bus Creator4/1 -> Bus Creator6/4  "wCMD"
  gripperCMD/2(REV) -> Bus Creator5/2  "rev"
  gripperCMD/3(BRK) -> Bus Creator5/3  "brk"
  gripperCMD/1(Duty) -> Bus Creator5/1  "duty"
  gripperPID/1 -> gripperCMD/1(Vcmd)  "gCMD"
  Break5/1 -> gripperCMD/2(Vbrk)
  Bus Creator5/1 -> Bus Creator6/6  "gCMD"
  Bus Creator/1 -> Bus Creator6/2  "bCMD"
  Bus Creator6/1 -> cmds/1
  ref Select/2 -> Sum1/2  "<bREF>"
  Constant1/1 -> Sum1/1
  fdbk/1 -> Signal Conditioning/1(fddk)
  Signal Conditioning/1(angles (rad)) -> Bus Selector/1
  Sum2/1 -> error/1
  ref Select/1 -> [q1_ref]  "<tREF>"
  ref Select/3 -> [q3_ref]  "<fREF>"
  ref Select/4 -> [q4_ref]  "<wREF>"
  ref Select/5 -> [q5_ref]  "<hREF>"
  ref Select/6 -> [q6_ref]  "<gREF>"
  Sum1/1 -> [q2_ref]
  [q1_ref] -> Sum2/1, turntablePID/1
  [q2_ref] -> bicepPID/1
  [q3_ref] -> forearmPID/1
  [q4_ref] -> wristPID/1
  [q6_ref] -> gripperPID/1
  Bus Selector/1 -> [q1_fdbk]  "<tAngle>"
  Bus Selector/2 -> [q2_fdbk]  "<bAngle>"
  Bus Selector/3 -> [q3_fdbk]  "<fAngle>"
  Bus Selector/4 -> [q4_fdbk]  "<wAngle>"
  Bus Selector/5 -> [q5_fdbk]  "<hAngle>"
  Bus Selector/6 -> [q6_fdbk]  "<gAngle>"
  [q1_fdbk] -> Sum2/2, turntablePID/2
  [q2_fdbk] -> bicepPID/2
  [q3_fdbk] -> forearmPID/2
  [q4_fdbk] -> wristPID/2
  [q5_fdbk] -> handPID/2
  [q5_ref] -> handPID/1
  [q6_fdbk] -> gripperPID/2

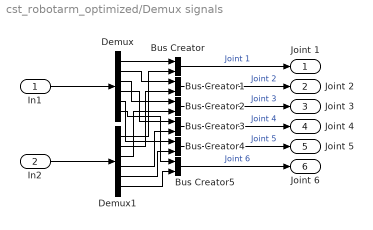
== system cst_robotarm_optimized/Demux signals ==
  In1 : Inport
  In2 : Inport  Port=2
  Bus Creator{,1..5} (6 alike) : BusCreator  Inputs=2
  Demux : Demux  Outputs=6
  Demux1 : Demux  Outputs=6
  Joint 1 : Outport
  Joint 2 : Outport  Port=2
  Joint 3 : Outport  Port=3
  Joint 4 : Outport  Port=4
  Joint 5 : Outport  Port=5
  Joint 6 : Outport  Port=6
  wires:
  Demux1/5 -> Bus Creator4/2
  Demux/1 -> Bus Creator/1
  Demux1/2 -> Bus Creator1/2
  Demux1/6 -> Bus Creator5/2
  Demux/3 -> Bus Creator2/1
  Demux1/1 -> Bus Creator/2
  Bus Creator/1 -> Joint 1/1  "Joint 1"
  Demux1/4 -> Bus Creator3/2
  Demux1/3 -> Bus Creator2/2
  Bus Creator3/1 -> Joint 4/1  "Joint 4"
  Demux/2 -> Bus Creator1/1
  Bus Creator1/1 -> Joint 2/1  "Joint 2"
  Bus Creator5/1 -> Joint 6/1  "Joint 6"
  In2/1 -> Demux1/1
  Bus Creator2/1 -> Joint 3/1  "Joint 3"
  Bus Creator4/1 -> Joint 5/1  "Joint 5"
  In1/1 -> Demux/1
  Demux/4 -> Bus Creator3/1
  Demux/5 -> Bus Creator4/1
  Demux/6 -> Bus Creator5/1

== system cst_robotarm_optimized/Reference Angle Test Vectors ==
  Bus Creator : BusCreator  Inputs=6
  Gain{,1..5} (6 alike) : Gain  Gain=pi/180
  Joint Angle Test Vectors : SignalEditorBlockLib/Signal Editor  FileName=dcst_robotarm_JointAngleSignalEditorData.mat  ActiveScenario=Two_Points_Test_1  ActiveSignal=Gripper Angle (deg)  IsBus=off  OutputBusObjectStr=Bus: BusObject  SampleTime=0  OutputAfterFinalValue=Extrapolation  Unit=inherit  PreserveSignalName=on  ApplySigPropsToAllScenarios=on  ApplySigPropsToAllSignals=off
  ref : Outport  VectorParamsAs1DForOutWhenUnconnected=off
  wires:
  Joint Angle Test Vectors/1 -> Gain/1
  Joint Angle Test Vectors/2 -> Gain1/1
  Joint Angle Test Vectors/3 -> Gain2/1
  Joint Angle Test Vectors/4 -> Gain3/1
  Joint Angle Test Vectors/5 -> Gain4/1
  Joint Angle Test Vectors/6 -> Gain5/1
  Bus Creator/1 -> ref/1
  Gain/1 -> Bus Creator/1  "tREF"
  Gain1/1 -> Bus Creator/2  "bREF"
  Gain2/1 -> Bus Creator/3  "fREF"
  Gain3/1 -> Bus Creator/4  "wREF"
  Gain4/1 -> Bus Creator/5  "hREF"
  Gain5/1 -> Bus Creator/6  "gREF"

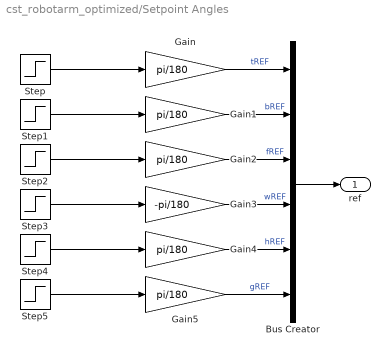
== system cst_robotarm_optimized/Setpoint Angles ==
  Bus Creator : BusCreator  Inputs=6
  Gain{,1..2,4..5} (5 alike) : Gain  Gain=pi/180
  Gain3 : Gain  Gain=-pi/180
  Step : Step  Time=0  After=joint1_ctrl  SampleTime=Ts
  Step1 : Step  Time=0  Before=90  After=joint2_ctrl  SampleTime=Ts
  Step2 : Step  Time=0  After=joint3_ctrl  SampleTime=Ts
  Step3 : Step  Time=0  After=joint4_ctrl  SampleTime=Ts
  Step4 : Step  Time=0  After=joint5_ctrl  SampleTime=Ts
  Step5 : Step  Time=0  After=joint6_ctrl  SampleTime=Ts
  ref : Outport  VectorParamsAs1DForOutWhenUnconnected=off
  wires:
  Gain5/1 -> Bus Creator/6  "gREF"
  Gain4/1 -> Bus Creator/5  "hREF"
  Gain3/1 -> Bus Creator/4  "wREF"
  Gain2/1 -> Bus Creator/3  "fREF"
  Gain1/1 -> Bus Creator/2  "bREF"
  Gain/1 -> Bus Creator/1  "tREF"
  Bus Creator/1 -> ref/1
  Step/1 -> Gain/1
  Step1/1 -> Gain1/1
  Step5/1 -> Gain5/1
  Step4/1 -> Gain4/1
  Step3/1 -> Gain3/1
  Step2/1 -> Gain2/1

== system cst_robotarm_optimized/Subsystem3 ==
